simulink model "example_simulink"  (R2023a)
settings: Solver=VariableStepAuto  StartTime=0.0  StopTime=10.0  RelTol=1e-3
settings Model: Creator=Martin  LastModifiedBy=Martin

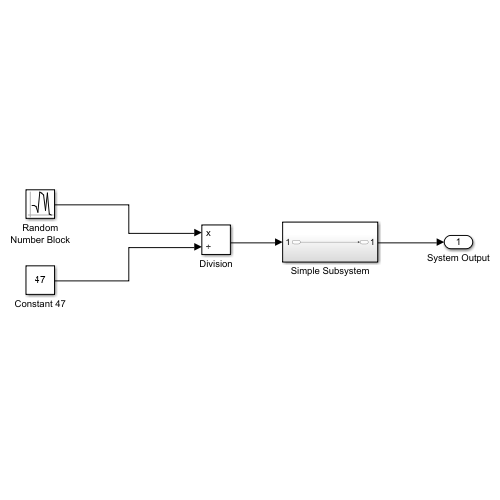
[thumbnail: Simulink's stored preview of the top-level diagram]
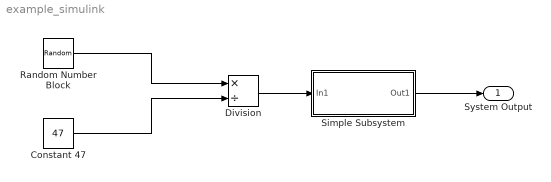
== system example_simulink ==
  Constant 47 : Constant  Value=47
  Division : Product  Inputs=*/
  Random Number Block : RandomNumber  SampleTime=0.1
  Simple Subsystem : Subsystem
  System Output : Outport
  wires:
  Division/1 -> Simple Subsystem/1(In1)
  Simple Subsystem/1(Out1) -> System Output/1
  Random Number Block/1 -> Division/1
  Constant 47/1 -> Division/2

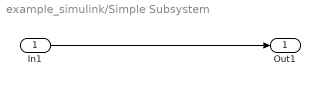
== system example_simulink/Simple Subsystem ==
  In1 : Inport
  Out1 : Outport
  wires:
  In1/1 -> Out1/1
